simulink model "real_time_test1"  (R2017b)
settings: Solver=VariableStepAuto  StartTime=0.0  StopTime=inf  RelTol=1e-3
libraries: sldrtlib x1
settings Model: Creator=mm395  LastModifiedBy=mm395

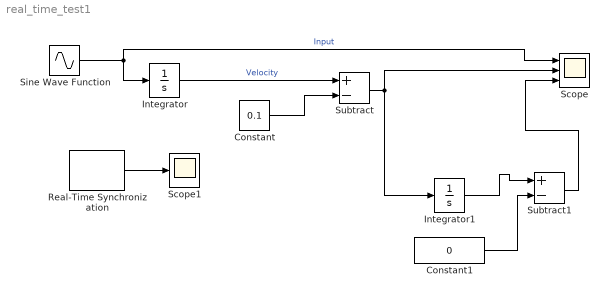
== system real_time_test1 ==
  Constant : Constant  Value=0.1
  Constant1 : Constant  Value=0
  Integrator : Integrator  ContinuousStateAttributes='velocity'
  Integrator1 : Integrator  ZeroCross=off  ContinuousStateAttributes='position'
  Real-Time Synchronization : sldrtlib/Real-Time Synchronization  SampleTime=0.01  MaxMissedTicks=100  ShowMissedTicks=on  YieldWhenWaiting=off
  Scope : Scope  NumInputPorts=3
  Scope1 : Scope
  Sine Wave Function : Sin  Frequency=10  SampleTime=0.01
  Subtract : Sum  Inputs=+-
  Subtract1 : Sum  Inputs=+-
  wires:
  Sine Wave Function/1 -> Integrator/1, Scope/1  "Input"
  Integrator/1 -> Subtract/1  "Velocity"
  Integrator1/1 -> Subtract1/1
  Subtract/1 -> Scope/2, Integrator1/1
  Constant/1 -> Subtract/2
  Constant1/1 -> Subtract1/2
  Subtract1/1 -> Scope/3
  Real-Time Synchronization/1 -> Scope1/1
